simulink model "prelim_FFT_blockFP"  (R2013a)
settings: Solver=ode45  StartTime=0.0  StopTime=10000  RelTol=1e-3
PostLoadFcn:
  | bps_model_init(gcs);
libraries: xbsIndex_r4 x41
settings Model: Creator=BEEcube  LastModifiedBy=rijesh
settings DataIOCC: SignalLoggingSaveFormat=ModelDataLogs
settings OptimizationCC: InlineParams=on  ExpressionDepthLimit=2147483647
settings DebuggingCC: FcnCallInpInsideContextMsg=UseLocalSettings
settings GRTTargetCC: CombineOutputUpdateFcns=off  GRTInterface=on

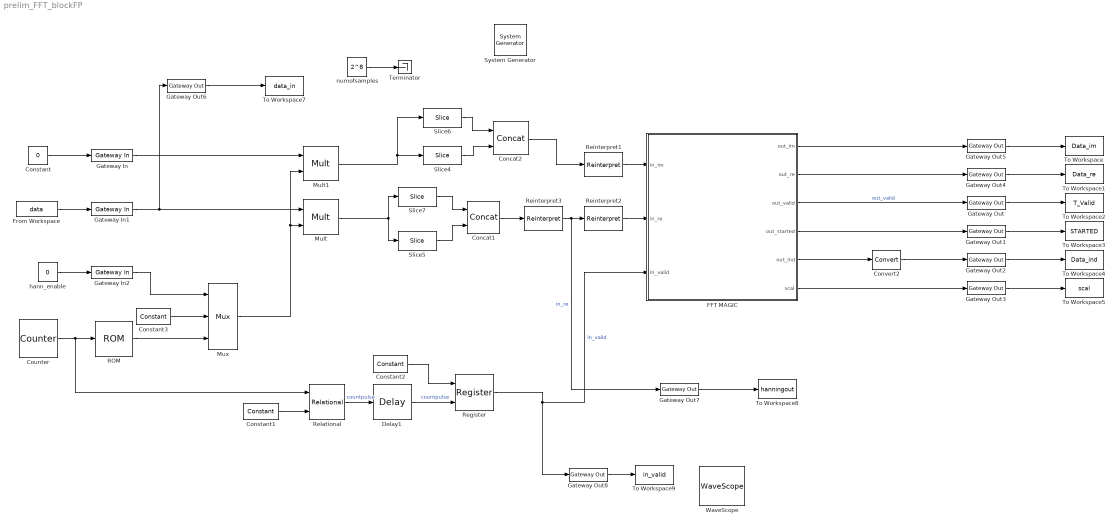
== system prelim_FFT_blockFP ==
  " System Generator" : xbsIndex_r4/ System Generator  Tag=genX  xilinxfamily=virtex6  part=xc6vsx475t  speed=-2  package=ff1759  synthesis_tool=XST  clock_wrapper=Clock Enables  directory=./prelim_FFT_blockFP/sysgen  proj_type=Project Navigator  Synth_file=XST Defaults  Impl_file=ISE Defaults  testbench=off  simulink_period=1  sysclk_period=4  dcm_input_clock_period=10  incr_netlist=off  trim_vbits=Everywhere in SubSystem  dbl_ovrd=According to Block Masks  core_generation=According to Block Masks  run_coregen=off  deprecated_control=off  eval_field=0  block_type=sysgen
  Concat1 : xbsIndex_r4/Concat  num_inputs=2  dbl_ovrd=off  block_type=concat
  Concat2 : xbsIndex_r4/Concat  num_inputs=2  dbl_ovrd=off  block_type=concat
  Constant : Constant  Value=0
  Constant1 : xbsIndex_r4/Constant  const=str2num(get_param('prelim_FFT_blockFP/numofsamples','value'))-1  gui_display_data_type=Fixed-point  arith_type=Unsigned  n_bits=log2(str2num(get_param('prelim_FFT_blockFP/numofsamples','value')))  bin_pt=0  preci_type=Single  exp_width=8  frac_width=24  explicit_period=off  period=1  equ=P=C  opselect=C  inp2=PCIN>>17  opr=+  inp1=P  carry=CIN  dbl_ovrd=off  block_type=constant
  Constant2 : xbsIndex_r4/Constant  const=1  gui_display_data_type=Boolean  arith_type=Boolean  n_bits=8  bin_pt=0  preci_type=Single  exp_width=8  frac_width=24  explicit_period=off  period=1  equ=P=C  opselect=C  inp2=PCIN>>17  opr=+  inp1=P  carry=CIN  dbl_ovrd=off  block_type=constant
  Constant3 : xbsIndex_r4/Constant  const=1  gui_display_data_type=Fixed-point  arith_type=Signed (2's comp)  n_bits=16  bin_pt=14  preci_type=Single  exp_width=8  frac_width=24  explicit_period=off  period=1  equ=P=C  opselect=C  inp2=PCIN>>17  opr=+  inp1=P  carry=CIN  dbl_ovrd=off  block_type=constant
  Convert2 : xbsIndex_r4/Convert  gui_display_data_type=Fixed-point  arith_type=Unsigned  n_bits=8  bin_pt=0  float_type=Double  exp_bits=8  fraction_bits=24  quantization=Truncate  overflow=Wrap  en=off  latency=0  dbl_ovrd=off  pipeline=off  block_type=convert
  Counter : xbsIndex_r4/Counter  cnt_type=Free Running  cnt_to=Inf  operation=Up  start_count=0  cnt_by_val=1  arith_type=Unsigned  n_bits=log2(str2num(get_param('prelim_FFT_blockFP/numofsamples','value')))  bin_pt=0  load_pin=off  rst=off  en=off  explicit_period=on  period=1  dbl_ovrd=off  use_behavioral_HDL=off  implementation=Fabric  block_type=counter
  Delay1 : xbsIndex_r4/Delay  rst=off  infoeditControl=Selection of Reset will increase slice count due to use of real FFs and instead of SRLs  en=off  latency=4  dbl_ovrd=off  reg_retiming=off  block_type=delay
  FFT MAGIC : Subsystem
  From Workspace : FromWorkspace  VariableName=data  SampleTime=0
  Gateway In : xbsIndex_r4/Gateway In  gui_display_data_type=Fixed-point  arith_type="Signed  (2's comp)"  n_bits=14  bin_pt=0  preci_type=Single  exp_width=8  frac_width=24  quantization="Round  (unbiased: +/- Inf)"  overflow=Saturate  period=1  dbl_ovrd=off  timing_constraint=None  locs_specified=off  LOCs={}  UseAsADC=off  ADCChannel='1'  inherit_from_input=off  hdl_port=on  block_type=gatewayin
  Gateway In1 : xbsIndex_r4/Gateway In  gui_display_data_type=Fixed-point  arith_type="Signed  (2's comp)"  n_bits=14  bin_pt=0  preci_type=Single  exp_width=8  frac_width=24  quantization="Round  (unbiased: +/- Inf)"  overflow=Saturate  period=1  dbl_ovrd=off  timing_constraint=None  locs_specified=off  LOCs={}  UseAsADC=off  ADCChannel='1'  inherit_from_input=off  hdl_port=on  block_type=gatewayin
  Gateway In2 : xbsIndex_r4/Gateway In  gui_display_data_type=Fixed-point  arith_type=Unsigned  n_bits=1  bin_pt=0  preci_type=Single  exp_width=8  frac_width=24  quantization="Round  (unbiased: +/- Inf)"  overflow=Saturate  period=1  dbl_ovrd=off  timing_constraint=None  locs_specified=off  LOCs={}  UseAsADC=off  ADCChannel='1'  inherit_from_input=off  hdl_port=on  block_type=gatewayin
  Gateway Out{,1..8} (9 alike) : xbsIndex_r4/Gateway Out  inherit_from_input=off  hdl_port=on  timing_constraint=None  locs_specified=off  LOCs={}  UseAsDAC=off  DACChannel='1'  block_type=gatewayout
  Mult : xbsIndex_r4/Mult  precision=Full  arith_type="Signed  (2's comp)"  n_bits=16  bin_pt=14  quantization=Truncate  overflow=Wrap  en=off  latency=3  dbl_ovrd=off  use_behavioral_HDL=off  opt=Speed  use_embedded=on  optimum_pipeline=off  pipeline=on  use_rpm=on  placement_style=Triangular  block_type=mult
  Mult1 : xbsIndex_r4/Mult  precision=Full  arith_type="Signed  (2's comp)"  n_bits=16  bin_pt=14  quantization=Truncate  overflow=Wrap  en=off  latency=3  dbl_ovrd=off  use_behavioral_HDL=off  opt=Speed  use_embedded=on  optimum_pipeline=off  pipeline=on  use_rpm=on  placement_style=Triangular  block_type=mult
  Mux : xbsIndex_r4/Mux  inputs=2  en=off  latency=0  precision=Full  arith_type=Unsigned  n_bits=16  bin_pt=14  quantization=Truncate  overflow=Wrap  dbl_ovrd=off  block_type=mux
  ROM : xbsIndex_r4/ROM  depth=str2num(get_param('prelim_FFT_blockFP/numofsamples','value'))  initVector=hann(str2num(get_param('prelim_FFT_blockFP/numofsamples','value')))  distributed_mem=Distributed memory  rst=off  init_reg=0  en=off  latency=1  gui_display_data_type=Fixed-point  arith_type="Signed  (2's comp)"  n_bits=16  bin_pt=14  preci_type=Single  exp_width=8  frac_width=24  dbl_ovrd=off  optimize=Area  use_rpm=on  block_type=sprom
  Register : xbsIndex_r4/Register  init=0  rst=off  en=on  dbl_ovrd=off  block_type=register
  Reinterpret1 : xbsIndex_r4/Reinterpret  force_arith_type=on  arith_type="Signed  (2's comp)"  force_bin_pt=on  bin_pt=13  block_type=reinterpret
  Reinterpret2 : xbsIndex_r4/Reinterpret  force_arith_type=on  arith_type="Signed  (2's comp)"  force_bin_pt=on  bin_pt=13  block_type=reinterpret
  Reinterpret3 : xbsIndex_r4/Reinterpret  force_arith_type=on  arith_type="Signed  (2's comp)"  force_bin_pt=on  bin_pt=0  block_type=reinterpret
  Relational : xbsIndex_r4/Relational  mode=a=b  en=off  latency=0  dbl_ovrd=off  block_type=relational
  Slice4 : xbsIndex_r4/Slice  nbits=13  boolean_output=off  mode=Lower Bit Location + Width  bit1=0  base1=MSB of Input  bit0=0  base0=Binary Point of Input  dbl_ovrd=off  block_type=slice
  Slice5 : xbsIndex_r4/Slice  nbits=13  boolean_output=off  mode=Lower Bit Location + Width  bit1=0  base1=MSB of Input  bit0=0  base0=Binary Point of Input  dbl_ovrd=off  block_type=slice
  Slice6 : xbsIndex_r4/Slice  nbits=1  boolean_output=off  mode=Upper Bit Location + Width  bit1=0  base1=MSB of Input  bit0=0  base0=Binary Point of Input  dbl_ovrd=off  block_type=slice
  Slice7 : xbsIndex_r4/Slice  nbits=1  boolean_output=off  mode=Upper Bit Location + Width  bit1=0  base1=MSB of Input  bit0=0  base0=Binary Point of Input  dbl_ovrd=off  block_type=slice
  Terminator : Terminator
  To Workspace : ToWorkspace  VariableName=Data_im  SampleTime=-1  SaveFormat=Timeseries
  To Workspace1 : ToWorkspace  VariableName=Data_re  SampleTime=-1  SaveFormat=Timeseries
  To Workspace2 : ToWorkspace  VariableName=T_Valid  SampleTime=-1  SaveFormat=Timeseries
  To Workspace3 : ToWorkspace  VariableName=STARTED  SampleTime=-1  SaveFormat=Timeseries
  To Workspace4 : ToWorkspace  VariableName=Data_ind  SampleTime=-1  SaveFormat=Timeseries
  To Workspace5 : ToWorkspace  VariableName=scal  SampleTime=-1  SaveFormat=Timeseries
  To Workspace7 : ToWorkspace  VariableName=data_in  SampleTime=-1  SaveFormat=Timeseries
  To Workspace8 : ToWorkspace  VariableName=hanningout  SampleTime=-1  SaveFormat=Timeseries
  To Workspace9 : ToWorkspace  VariableName=in_valid  SampleTime=-1  SaveFormat=Timeseries
  WaveScope : xbsIndex_r4/WaveScope  block_type=wavescope
  hann_enable : Constant  Value=0
  numofsamples : Constant  Value=2^8
  wires:
  From Workspace/1 -> Gateway In1/1
  Constant/1 -> Gateway In/1
  Gateway Out6/1 -> To Workspace7/1
  Mult1/1 -> Slice6/1, Slice4/1
  Gateway In1/1 -> Mult/1, Gateway Out6/1
  Register/1 -> Gateway Out8/1, FFT MAGIC/3(in_valid)  "in_valid"
  FFT MAGIC/5(out_ind) -> Convert2/1
  FFT MAGIC/4(out_started) -> Gateway Out1/1
  FFT MAGIC/3(out_valid) -> Gateway Out/1  "out_valid"
  Gateway Out5/1 -> To Workspace/1
  Gateway Out4/1 -> To Workspace1/1
  Gateway Out/1 -> To Workspace2/1
  Gateway Out1/1 -> To Workspace3/1
  Gateway Out2/1 -> To Workspace4/1
  FFT MAGIC/2(out_re) -> Gateway Out4/1
  FFT MAGIC/1(out_im) -> Gateway Out5/1
  Convert2/1 -> Gateway Out2/1
  FFT MAGIC/6(scal) -> Gateway Out3/1
  Gateway Out3/1 -> To Workspace5/1
  Mux/1 -> Mult1/2, Mult/2
  Mult/1 -> Slice7/1, Slice5/1
  Counter/1 -> Relational/1, ROM/1
  Gateway In/1 -> Mult1/1
  Reinterpret1/1 -> FFT MAGIC/1(in_im)
  Reinterpret2/1 -> FFT MAGIC/2(in_re)
  Concat2/1 -> Reinterpret1/1
  Constant1/1 -> Relational/2
  Gateway Out7/1 -> To Workspace8/1
  Slice5/1 -> Concat1/2
  Slice7/1 -> Concat1/1
  Slice4/1 -> Concat2/2
  Slice6/1 -> Concat2/1
  Reinterpret3/1 -> Gateway Out7/1, Reinterpret2/1  "in_re"
  Concat1/1 -> Reinterpret3/1
  Gateway Out8/1 -> To Workspace9/1
  Delay1/1 -> Register/2  "countpulse"
  Constant2/1 -> Register/1
  Relational/1 -> Delay1/1  "countpulse"
  numofsamples/1 -> Terminator/1
  ROM/1 -> Mux/3
  Constant3/1 -> Mux/2
  hann_enable/1 -> Gateway In2/1
  Gateway In2/1 -> Mux/1

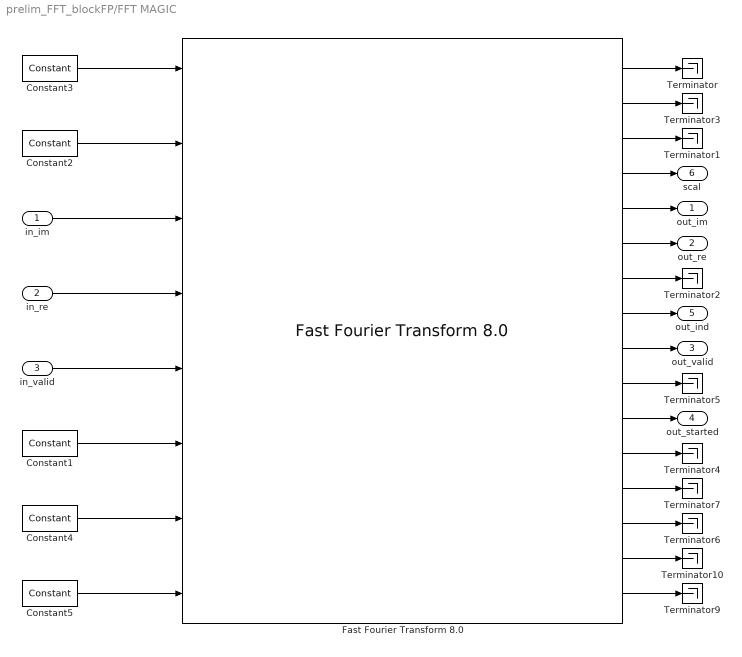
== system prelim_FFT_blockFP/FFT MAGIC ==
  in_im : Inport
  in_re : Inport  Port=2
  in_valid : Inport  Port=3
  Constant1 : xbsIndex_r4/Constant  const=0  gui_display_data_type=Boolean  arith_type=Boolean  n_bits=1  bin_pt=0  preci_type=Single  exp_width=8  frac_width=24  explicit_period=off  period=1  equ=P=C  opselect=C  inp2=PCIN>>17  opr=+  inp1=P  carry=CIN  dbl_ovrd=off  block_type=constant
  Constant2 : xbsIndex_r4/Constant  const=1  gui_display_data_type=Boolean  arith_type=Boolean  n_bits=1  bin_pt=0  preci_type=Single  exp_width=8  frac_width=24  explicit_period=off  period=1  equ=P=C  opselect=C  inp2=PCIN>>17  opr=+  inp1=P  carry=CIN  dbl_ovrd=off  block_type=constant
  Constant3 : xbsIndex_r4/Constant  const=1  gui_display_data_type=Fixed-point  arith_type=Unsigned  n_bits=1  bin_pt=0  preci_type=Single  exp_width=8  frac_width=24  explicit_period=off  period=1  equ=P=C  opselect=C  inp2=PCIN>>17  opr=+  inp1=P  carry=CIN  dbl_ovrd=off  block_type=constant
  Constant4 : xbsIndex_r4/Constant  const=1  gui_display_data_type=Boolean  arith_type=Boolean  n_bits=1  bin_pt=0  preci_type=Single  exp_width=8  frac_width=24  explicit_period=off  period=1  equ=P=C  opselect=C  inp2=PCIN>>17  opr=+  inp1=P  carry=CIN  dbl_ovrd=off  block_type=constant
  Constant5 : xbsIndex_r4/Constant  const=1  gui_display_data_type=Boolean  arith_type=Boolean  n_bits=1  bin_pt=0  preci_type=Single  exp_width=8  frac_width=24  explicit_period=off  period=1  equ=P=C  opselect=C  inp2=PCIN>>17  opr=+  inp1=P  carry=CIN  dbl_ovrd=off  block_type=constant
  "Fast Fourier Transform 8.0 " : xbsIndex_r4/Fast Fourier Transform 8.0   transform_length=256  target_clock_frequency=100  target_data_throughput=50  implementation_options=pipelined_streaming_io  run_time_configurable_transform_length=off  phase_factor_width=19  scaling_options=block_floating_point  rounding_modes=truncation  aclken=off  aresetn=off  cyclic_prefix_insertion=off  output_ordering=natural_order  throttle_scheme=nonrealtime  xk_index=on  ovflo=off  trim_axipin_name=off  memory_options_data=distributed_ram  memory_options_phase_factors=distributed_ram  number_of_stages_using_block_ram_for_data_and_phase_factors=0  memory_options_reorder=block_ram  memory_options_hybrid=off  complex_mult_type=use_mults_resources  butterfly_type=use_luts  channels=1  input_ordering=natural_order  input_width=16  ip_name=Fast Fourier Transform  ip_version=8.0  dsptool_ready=true  ipcore_usecache=true  ipcore_useipmodelcache=true  wrapper_available=true  port_translation_map={ 'aclken' => 'en', 'aresetn' => 'rst'}  block_type=xfft_v8_0
  Terminator{,1..7,9..10} (10 alike) : Terminator
  out_im : Outport
  out_re : Outport  Port=2
  out_valid : Outport  Port=3
  out_started : Outport  Port=4
  out_ind : Outport  Port=5
  scal : Outport  Port=6
  wires:
  "Fast Fourier Transform 8.0 "/11 -> out_started/1
  Constant1/1 -> "Fast Fourier Transform 8.0 "/6
  "Fast Fourier Transform 8.0 "/3 -> Terminator1/1
  in_im/1 -> "Fast Fourier Transform 8.0 "/3
  in_re/1 -> "Fast Fourier Transform 8.0 "/4
  "Fast Fourier Transform 8.0 "/12 -> Terminator4/1
  "Fast Fourier Transform 8.0 "/6 -> out_re/1
  "Fast Fourier Transform 8.0 "/1 -> Terminator/1
  "Fast Fourier Transform 8.0 "/10 -> Terminator5/1
  "Fast Fourier Transform 8.0 "/7 -> Terminator2/1
  "Fast Fourier Transform 8.0 "/9 -> out_valid/1
  in_valid/1 -> "Fast Fourier Transform 8.0 "/5
  "Fast Fourier Transform 8.0 "/5 -> out_im/1
  "Fast Fourier Transform 8.0 "/2 -> Terminator3/1
  "Fast Fourier Transform 8.0 "/8 -> out_ind/1
  Constant2/1 -> "Fast Fourier Transform 8.0 "/2
  Constant3/1 -> "Fast Fourier Transform 8.0 "/1
  "Fast Fourier Transform 8.0 "/14 -> Terminator6/1
  "Fast Fourier Transform 8.0 "/13 -> Terminator7/1
  "Fast Fourier Transform 8.0 "/4 -> scal/1
  "Fast Fourier Transform 8.0 "/16 -> Terminator9/1
  "Fast Fourier Transform 8.0 "/15 -> Terminator10/1
  Constant4/1 -> "Fast Fourier Transform 8.0 "/7
  Constant5/1 -> "Fast Fourier Transform 8.0 "/8
